simulink model "photocurrent"  (Simulink 7.5)
settings: Solver=ode45  StartTime=0.0  StopTime=10.0  RelTol=1e-3
settings Model: Creator=dell  LastModifiedBy=dell

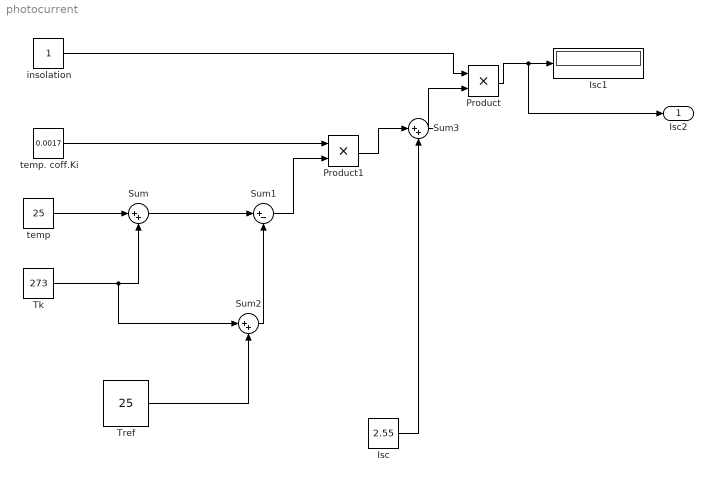
== system photocurrent ==
  Isc : Constant  Value=2.55  OutDataType=fixdt(1, 16)  OutScaling=2^0
  Isc1 : Display
  Product : Product  OutDataType=fixdt(1, 16)  OutScaling=2^0  RndMeth=Zero
  Product1 : Product  OutDataType=fixdt(1, 16)  OutScaling=2^0  RndMeth=Zero
  Sum : Sum  Inputs=|++  OutDataType=fixdt(1, 16)  OutScaling=2^0
  Sum1 : Sum  Inputs=|+-  OutDataType=fixdt(1, 16)  OutScaling=2^0
  Sum2 : Sum  Inputs=|++  OutDataType=fixdt(1, 16)  OutScaling=2^0
  Sum3 : Sum  Inputs=|++  OutDataType=fixdt(1, 16)  OutScaling=2^0
  Tk : Constant  Value=273  OutDataType=fixdt(1, 16)  OutScaling=2^0
  Tref : Constant  Value=25  OutDataType=fixdt(1, 16)  OutScaling=2^0
  insolation : Constant  OutDataType=fixdt(1, 16)  OutScaling=2^0
  temp : Constant  Value=25  OutDataType=fixdt(1, 16)  OutScaling=2^0
  temp. coff.Ki : Constant  Value=0.0017  OutDataType=fixdt(1, 16)  OutScaling=2^0
  Isc2 : Outport  OutDataType=fixdt(1, 16)  OutScaling=2^0
  wires:
  insolation/1 -> Product/1
  Product/1 -> Isc1/1, Isc2/1
  temp. coff.Ki/1 -> Product1/1
  temp/1 -> Sum/1
  Tk/1 -> Sum/2, Sum2/1
  Sum/1 -> Sum1/1
  Tref/1 -> Sum2/2
  Sum2/1 -> Sum1/2
  Sum1/1 -> Product1/2
  Product1/1 -> Sum3/1
  Isc/1 -> Sum3/2
  Sum3/1 -> Product/2
